simulink model "sampleModel84"  (Simulink 9.1)
settings: Solver=VariableStepAuto  StartTime=0.0  StopTime=10.0  RelTol=1e-3
undefined symbols (not defined in the file): DiscIntNeverNeededParam, Newton, Raphson
libraries: simulink x55
(part 2 of 2)

== system sampleModel84/cfblk150 ==
  cfblk1 : Inport
  cfblk8 : Inport  Port=2
  Action Port : ActionPort  ActionType=then
  cfblk3 : simulink/Continuous/PID Controller  Controller=PID  TimeDomain=Discrete-time  SampleTime=-1  IntegratorMethod=Forward Euler  FilterMethod=Forward Euler  Form=Parallel  UseFilter=on  ControllerParametersSource=internal  P=1  I=1  D=0  N=100  InitialConditionSource=internal  InitialConditionForIntegrator=0  InitialConditionForFilter=0  ExternalReset=none  LimitOutput=off  UpperSaturationLimit=inf  LowerSaturationLimit=-inf  LinearizeAsGain=off  AntiWindupMode=none  Kb=1  TrackingMode=off  Kt=1  PParamMin=[]  PParamMax=[]  IParamMin=[]  IParamMax=[]  DParamMin=[]  DParamMax=[]  NParamMin=[]  NParamMax=[]  KbParamMin=[]  KbParamMax=[]  KtParamMin=[]  KtParamMax=[]  POutMin=[]  POutMax=[]  IOutMin=[]  IOutMax=[]  DOutMin=[]  DOutMax=[]  NOutMin=[]  NOutMax=[]  KbOutMin=[]  KbOutMax=[]  KtOutMin=[]  KtOutMax=[]  IntegratorOutMin=[]  IntegratorOutMax=[]  FilterOutMin=[]  FilterOutMax=[]  SumOutMin=[]  SumOutMax=[]  SumI1OutMin=[]  SumI1OutMax=[]  SumI2OutMin=[]  SumI2OutMax=[]  SumI3OutMin=[]  SumI3OutMax=[]  SumDOutMin=[]  SumDOutMax=[]  SaturationOutMin=[]  SaturationOutMax=[]  IntegratorContinuousStateAttributes=''  IntegratorStateMustResolveToSignalObject=off  IntegratorRTWStateStorageClass=Auto  FilterContinuousStateAttributes=''  FilterStateMustResolveToSignalObject=off  FilterRTWStateStorageClass=Auto  DifferentiatorICPrevScaledInput=0  DifferentiatorOutMin=[]  DifferentiatorOutMax=[]  FilterDiffOutCoefMin=[]  FilterDiffOutCoefMax=[]  SumDenOutMin=[]  SumDenOutMax=[]  SumNumOutMin=[]  SumNumOutMax=[]  ReciprocalOutMin=[]  ReciprocalOutMax=[]  DivideOutMin=[]  DivideOutMax=[]  TunerSelectOption=Transfer Function Based (PID Tuner App)
  cfblk4 : Trigonometry
  cfblk5 : UnaryMinus
  cfblk6 : Sqrt  Operator=rSqrt  AlgorithmType=Newton-Raphson  SaturateOnIntegerOverflow=on
  cfblk7 : Subsystem
  cfblk2 : Outport
  cfblk9 : Outport  Port=2
  cfblk10 : Outport  Port=3
  wires:
  cfblk1/1 -> cfblk5/1
  cfblk4/1 -> cfblk3/1, cfblk9/1
  cfblk5/1 -> cfblk4/1
  cfblk8/1 -> cfblk2/1
  cfblk6/1 -> cfblk10/1
  cfblk7/1(cfblk2) -> cfblk6/1
  cfblk3/1 -> cfblk7/1(cfblk1)

== system sampleModel84/cfblk151 ==
  cfblk1 : Inport
  cfblk8 : Inport  Port=2
  cfblk9 : Inport  Port=3
  Action Port : ActionPort  ActionType=else
  cfblk10 : Delay
  cfblk3 : Delay  DelayLengthSource=Input port
      settings: InputPortMap=u0,p1
  cfblk4 : simulink/Discrete/Transfer Fcn Lead or Lag  PoleZ=0.95  ZeroZ=0.75  ICPrevOutput=0.0  ICPrevInput=0.0  DoSatur=off
      settings: SourceProductName=Simulink  SourceProductBaseCode=SL
  cfblk5 : DotProduct  InputSameDT=on  OutDataTypeStr=Inherit: Inherit via internal rule
  cfblk6 : Bias  Bias=[-271351723.485476]
  cfblk7 : Subsystem
  cfblk2 : Outport
  wires:
  cfblk9/1 -> cfblk4/1
  cfblk3/1 -> cfblk7/1(cfblk1)
  cfblk1/1 -> cfblk3/1
  cfblk6/1 -> cfblk2/1
  cfblk7/1(cfblk2) -> cfblk5/1
  cfblk8/1 -> cfblk5/2
  cfblk4/1 -> cfblk6/1
  cfblk5/1 -> cfblk10/1
  cfblk10/1 -> cfblk3/2

== system sampleModel84/cfblk98 ==
  cfblk1 : Inport
  cfblk2 : Outport
  wires:
  cfblk1/1 -> cfblk2/1

== system sampleModel84/cfblk99 ==
  cfblk1 : Inport
  cfblk2 : Outport
  wires:
  cfblk1/1 -> cfblk2/1

== system sampleModel84/cfblk134/cfblk11 ==
  cfblk1 : Inport
  cfblk2 : Outport
  wires:
  cfblk1/1 -> cfblk2/1

== system sampleModel84/cfblk134/cfblk12 ==
  cfblk1 : Inport
  cfblk2 : Outport
  wires:
  cfblk1/1 -> cfblk2/1

== system sampleModel84/cfblk134/cfblk13 ==
  cfblk1 : Inport
  cfblk2 : Outport
  wires:
  cfblk1/1 -> cfblk2/1

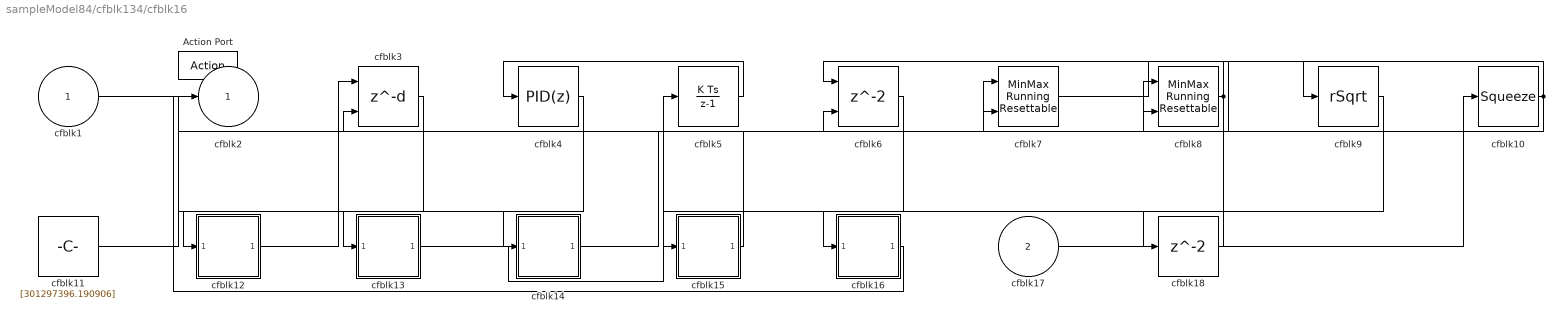
== system sampleModel84/cfblk134/cfblk16 ==
  cfblk1 : Inport
  cfblk17 : Inport  Port=2
  Action Port : ActionPort  ActionType=then
  cfblk10 : Squeeze
  cfblk11 : Constant  Value=[301297396.190906]  SampleTime=1
  cfblk12 : Subsystem
  cfblk13 : Subsystem
  cfblk14 : Subsystem
  cfblk15 : Subsystem
  cfblk16 : Subsystem
  cfblk18 : Delay
  cfblk3 : Delay  DelayLengthSource=Input port
      settings: InputPortMap=u0,p1
  cfblk4 : simulink/Continuous/PID Controller  Controller=PID  TimeDomain=Discrete-time  SampleTime=-1  IntegratorMethod=Forward Euler  FilterMethod=Forward Euler  Form=Parallel  UseFilter=on  ControllerParametersSource=internal  P=1  I=1  D=0  N=100  InitialConditionSource=internal  InitialConditionForIntegrator=0  InitialConditionForFilter=0  ExternalReset=none  LimitOutput=off  UpperSaturationLimit=inf  LowerSaturationLimit=-inf  LinearizeAsGain=off  AntiWindupMode=none  Kb=1  TrackingMode=off  Kt=1  PParamMin=[]  PParamMax=[]  IParamMin=[]  IParamMax=[]  DParamMin=[]  DParamMax=[]  NParamMin=[]  NParamMax=[]  KbParamMin=[]  KbParamMax=[]  KtParamMin=[]  KtParamMax=[]  POutMin=[]  POutMax=[]  IOutMin=[]  IOutMax=[]  DOutMin=[]  DOutMax=[]  NOutMin=[]  NOutMax=[]  KbOutMin=[]  KbOutMax=[]  KtOutMin=[]  KtOutMax=[]  IntegratorOutMin=[]  IntegratorOutMax=[]  FilterOutMin=[]  FilterOutMax=[]  SumOutMin=[]  SumOutMax=[]  SumI1OutMin=[]  SumI1OutMax=[]  SumI2OutMin=[]  SumI2OutMax=[]  SumI3OutMin=[]  SumI3OutMax=[]  SumDOutMin=[]  SumDOutMax=[]  SaturationOutMin=[]  SaturationOutMax=[]  IntegratorContinuousStateAttributes=''  IntegratorStateMustResolveToSignalObject=off  IntegratorRTWStateStorageClass=Auto  FilterContinuousStateAttributes=''  FilterStateMustResolveToSignalObject=off  FilterRTWStateStorageClass=Auto  DifferentiatorICPrevScaledInput=0  DifferentiatorOutMin=[]  DifferentiatorOutMax=[]  FilterDiffOutCoefMin=[]  FilterDiffOutCoefMax=[]  SumDenOutMin=[]  SumDenOutMax=[]  SumNumOutMin=[]  SumNumOutMax=[]  ReciprocalOutMin=[]  ReciprocalOutMax=[]  DivideOutMin=[]  DivideOutMax=[]  TunerSelectOption=Transfer Function Based (PID Tuner App)
  cfblk5 : DiscreteIntegrator  SampleTime=-1  ICPrevOutput=DiscIntNeverNeededParam  ICPrevScaledInput=DiscIntNeverNeededParam
  cfblk6 : Delay  ShowEnablePort=on
      settings: InputPortMap=u0,e6
  cfblk7 : simulink/Math Operations/MinMax Running Resettable  Function=min  vinit=0.0
  cfblk8 : simulink/Math Operations/MinMax Running Resettable  Function=min  vinit=0.0
  cfblk9 : Sqrt  Operator=rSqrt  AlgorithmType=Newton-Raphson  SaturateOnIntegerOverflow=on
  cfblk2 : Outport
  wires:
  cfblk4/1 -> cfblk12/1(cfblk1)
  cfblk13/1(cfblk2) -> cfblk5/1
  cfblk16/1(cfblk2) -> cfblk2/1
  cfblk9/1 -> cfblk15/1(cfblk1)
  cfblk8/1 -> cfblk6/1, cfblk18/1
  cfblk15/1(cfblk2) -> cfblk3/2
  cfblk1/1 -> cfblk14/1(cfblk1)
  cfblk10/1 -> cfblk7/1, cfblk6/2
  cfblk7/1 -> cfblk9/1
  cfblk3/1 -> cfblk13/1(cfblk1)
  cfblk17/1 -> cfblk10/1
  cfblk5/1 -> cfblk4/1
  cfblk14/1(cfblk2) -> cfblk7/2
  cfblk6/1 -> cfblk16/1(cfblk1)
  cfblk11/1 -> cfblk8/1
  cfblk12/1(cfblk2) -> cfblk8/2
  cfblk18/1 -> cfblk3/1

== system sampleModel84/cfblk134/cfblk17 ==
  cfblk1 : Inport
  cfblk8 : Inport  Port=2
  cfblk9 : Inport  Port=3
  Action Port : ActionPort  ActionType=else
  cfblk3 : simulink/Discrete/Transfer Fcn Real Zero  ZeroZ=0.75  ICPrevInput=0.0  DoSatur=off
      settings: SourceProductName=Simulink  SourceProductBaseCode=SL
  cfblk4 : Reshape
  cfblk5 : MinMax  Function=max  Inputs=3
  cfblk6 : Assignment  DiagnosticForDimensions=Warning  IndexOptions=Index vector (dialog)  Indices=1  OutputSizes=1
  cfblk7 : Polyval  Coefs=[ +2.081618890e-019, -1.441693666e-014, +4.719686976e-010, -8.536869453e-006, +1.621573104e-001, -8.087801117e+001 ]
  cfblk2 : Outport
  wires:
  cfblk1/1 -> cfblk3/1
  cfblk7/1 -> cfblk6/1
  cfblk8/1 -> cfblk4/1, cfblk5/3
  cfblk9/1 -> cfblk7/1
  cfblk3/1 -> cfblk6/2
  cfblk6/1 -> cfblk5/1
  cfblk4/1 -> cfblk2/1, cfblk5/2

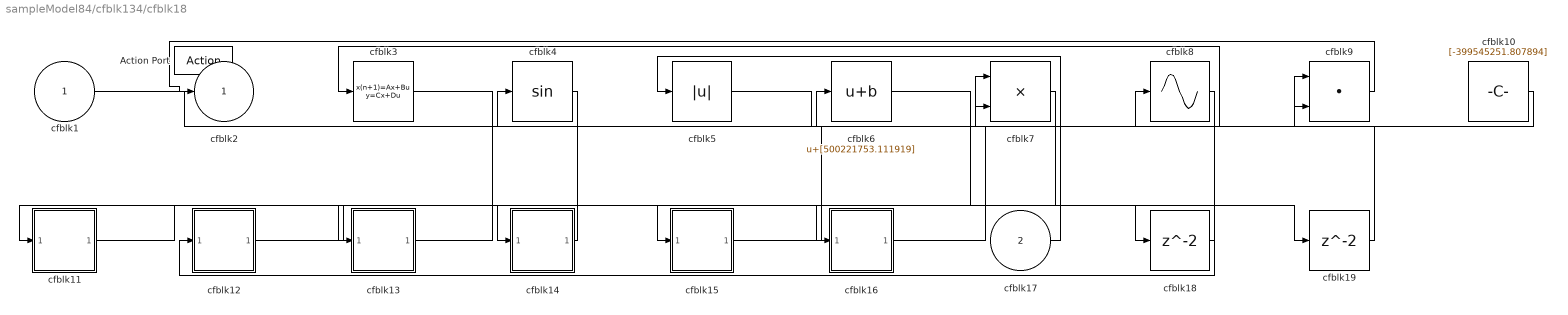
== system sampleModel84/cfblk134/cfblk18 ==
  cfblk1 : Inport
  cfblk17 : Inport  Port=2
  Action Port : ActionPort  ActionType=then
  cfblk10 : Constant  Value=[-399545251.807894]  SampleTime=1
  cfblk11 : Subsystem
  cfblk12 : Subsystem
  cfblk13 : Subsystem
  cfblk14 : Subsystem
  cfblk15 : Subsystem
  cfblk16 : Subsystem
  cfblk18 : Delay
  cfblk19 : Delay
  cfblk3 : DiscreteStateSpace  SampleTime=-1
  cfblk4 : Trigonometry
  cfblk5 : Abs
  cfblk6 : Bias  Bias=[500221753.111919]
  cfblk7 : Product  Inputs=**
  cfblk8 : Sin  TimeSource=Use external signal  SampleTime=0
  cfblk9 : DotProduct  InputSameDT=on  OutDataTypeStr=Inherit: Inherit via internal rule
  cfblk2 : Outport
  wires:
  cfblk1/1 -> cfblk7/1
  cfblk7/1 -> cfblk15/1(cfblk1)
  cfblk17/1 -> cfblk5/1
  cfblk8/1 -> cfblk12/1(cfblk1)
  cfblk12/1(cfblk2) -> cfblk14/1(cfblk1)
  cfblk9/1 -> cfblk2/1
  cfblk15/1(cfblk2) -> cfblk8/1
  cfblk10/1 -> cfblk3/1
  cfblk3/1 -> cfblk16/1(cfblk1)
  cfblk14/1(cfblk2) -> cfblk11/1(cfblk1)
  cfblk13/1(cfblk2) -> cfblk6/1
  cfblk4/1 -> cfblk13/1(cfblk1)
  cfblk16/1(cfblk2) -> cfblk9/1
  cfblk5/1 -> cfblk9/2
  cfblk11/1(cfblk2) -> cfblk18/1
  cfblk18/1 -> cfblk7/2
  cfblk6/1 -> cfblk19/1
  cfblk19/1 -> cfblk4/1

== system sampleModel84/cfblk134/cfblk19 ==
  cfblk1 : Inport
  Action Port : ActionPort  ActionType=else
  cfblk10 : Subsystem
  cfblk12 : Delay
  cfblk3 : simulink/Discrete/Difference  ICPrevInput=0.0  OutMin=[]  OutMax=[]  OutDataTypeStr=Inherit: Inherit via back propagation  OutDataType=fixdt(1, 16)  OutScaling=2^-10  DoSatur=off
  cfblk4 : simulink/Discrete/Transfer Fcn Real Zero  ZeroZ=0.75  ICPrevInput=0.0  DoSatur=off
      settings: SourceProductName=Simulink  SourceProductBaseCode=SL
  cfblk5 : Reshape
  cfblk6 : Polyval  Coefs=[ +2.081618890e-019, -1.441693666e-014, +4.719686976e-010, -8.536869453e-006, +1.621573104e-001, -8.087801117e+001 ]
  cfblk7 : Constant  Value=[-872675148.668030]  SampleTime=1
  cfblk8 : Subsystem
  cfblk9 : Subsystem
  cfblk2 : Outport
  cfblk11 : Outport  Port=2
  wires:
  cfblk5/1 -> cfblk8/1(cfblk1)
  cfblk6/1 -> cfblk9/1(cfblk1)
  cfblk1/1 -> cfblk3/1
  cfblk10/1(cfblk2) -> cfblk5/1
  cfblk8/1(cfblk2) -> cfblk11/1
  cfblk7/1 -> cfblk2/1
  cfblk4/1 -> cfblk10/1(cfblk1)
  cfblk3/1 -> cfblk4/1
  cfblk9/1(cfblk2) -> cfblk12/1
  cfblk12/1 -> cfblk6/1

== system sampleModel84/cfblk135/cfblk9 ==
  cfblk1 : Inport
  cfblk2 : Outport
  wires:
  cfblk1/1 -> cfblk2/1

== system sampleModel84/cfblk136/cfblk10 ==
  cfblk1 : Inport
  cfblk2 : Outport
  wires:
  cfblk1/1 -> cfblk2/1

== system sampleModel84/cfblk136/cfblk8 ==
  cfblk1 : Inport
  cfblk2 : Outport
  wires:
  cfblk1/1 -> cfblk2/1

== system sampleModel84/cfblk136/cfblk9 ==
  cfblk1 : Inport
  cfblk2 : Outport
  wires:
  cfblk1/1 -> cfblk2/1

== system sampleModel84/cfblk138/cfblk10 ==
  cfblk1 : Inport
  cfblk2 : Outport
  wires:
  cfblk1/1 -> cfblk2/1

== system sampleModel84/cfblk138/cfblk8 ==
  cfblk1 : Inport
  cfblk2 : Outport
  wires:
  cfblk1/1 -> cfblk2/1

== system sampleModel84/cfblk138/cfblk9 ==
  cfblk1 : Inport
  cfblk2 : Outport
  wires:
  cfblk1/1 -> cfblk2/1

== system sampleModel84/cfblk139/cfblk10 ==
  cfblk1 : Inport
  cfblk2 : Outport
  wires:
  cfblk1/1 -> cfblk2/1

== system sampleModel84/cfblk139/cfblk13 ==
  cfblk1 : Inport
  cfblk11 : Inport  Port=2
  cfblk12 : Inport  Port=3
  cfblk13 : Inport  Port=4
  cfblk14 : Inport  Port=5
  Action Port : ActionPort  ActionType=then
  cfblk10 : Subsystem
  cfblk3 : DiscreteTransferFcn
  cfblk4 : Squeeze
  cfblk5 : Sum  Inputs=+-
  cfblk6 : Sum  Inputs=+-
  cfblk7 : Sum  Inputs=|++
  cfblk8 : Product  Inputs=**
  cfblk9 : Constant  Value=[-663658281.904295]  SampleTime=1
  cfblk2 : Outport
  wires:
  cfblk1/1 -> cfblk2/1
  cfblk8/1 -> cfblk10/1(cfblk1)
  cfblk10/1(cfblk2) -> cfblk4/1
  cfblk3/1 -> cfblk7/1
  cfblk4/1 -> cfblk5/1
  cfblk11/1 -> cfblk6/1
  cfblk14/1 -> cfblk3/1
  cfblk6/1 -> cfblk7/2
  cfblk12/1 -> cfblk6/2
  cfblk7/1 -> cfblk8/1
  cfblk9/1 -> cfblk8/2
  cfblk13/1 -> cfblk5/2

== system sampleModel84/cfblk139/cfblk14 ==
  cfblk1 : Inport
  cfblk11 : Inport  Port=2
  cfblk12 : Inport  Port=3
  Action Port : ActionPort  ActionType=else
  cfblk10 : Subsystem
  cfblk3 : simulink/Discrete/Difference  ICPrevInput=0.0  OutMin=[]  OutMax=[]  OutDataTypeStr=Inherit: Inherit via back propagation  OutDataType=fixdt(1, 16)  OutScaling=2^-10  DoSatur=off
  cfblk4 : DiscreteStateSpace  SampleTime=-1
  cfblk5 : simulink/Discrete/Difference  ICPrevInput=0.0  OutMin=[]  OutMax=[]  OutDataTypeStr=Inherit: Inherit via back propagation  OutDataType=fixdt(1, 16)  OutScaling=2^-10  DoSatur=off
  cfblk6 : Math  Operator=conj  SaturateOnIntegerOverflow=on
  cfblk7 : Sum  Inputs=+
  cfblk8 : Constant  Value=[-583417160.658868]  SampleTime=1
  cfblk9 : Subsystem
  cfblk2 : Outport
  wires:
  cfblk1/1 -> cfblk9/1(cfblk1)
  cfblk10/1(cfblk2) -> cfblk5/1
  cfblk9/1(cfblk2) -> cfblk10/1(cfblk1)
  cfblk12/1 -> cfblk2/1
  cfblk8/1 -> cfblk6/1
  cfblk6/1 -> cfblk3/1
  cfblk3/1 -> cfblk7/1
  cfblk11/1 -> cfblk4/1

== system sampleModel84/cfblk139/cfblk8 ==
  cfblk1 : Inport
  cfblk2 : Outport
  wires:
  cfblk1/1 -> cfblk2/1

== system sampleModel84/cfblk139/cfblk9 ==
  cfblk1 : Inport
  cfblk2 : Outport
  wires:
  cfblk1/1 -> cfblk2/1

== system sampleModel84/cfblk140/cfblk11 ==
  cfblk1 : Inport
  cfblk2 : Outport
  wires:
  cfblk1/1 -> cfblk2/1

== system sampleModel84/cfblk140/cfblk12 ==
  cfblk1 : Inport
  cfblk2 : Outport
  wires:
  cfblk1/1 -> cfblk2/1

== system sampleModel84/cfblk140/cfblk13 ==
  cfblk1 : Inport
  cfblk2 : Outport
  wires:
  cfblk1/1 -> cfblk2/1

== system sampleModel84/cfblk140/cfblk14 ==
  cfblk1 : Inport
  cfblk2 : Outport
  wires:
  cfblk1/1 -> cfblk2/1

== system sampleModel84/cfblk141/cfblk11 ==
  cfblk1 : Inport
  cfblk2 : Outport
  wires:
  cfblk1/1 -> cfblk2/1

== system sampleModel84/cfblk141/cfblk12 ==
  cfblk1 : Inport
  cfblk2 : Outport
  wires:
  cfblk1/1 -> cfblk2/1

== system sampleModel84/cfblk141/cfblk13 ==
  cfblk1 : Inport
  cfblk2 : Outport
  wires:
  cfblk1/1 -> cfblk2/1

== system sampleModel84/cfblk141/cfblk14 ==
  cfblk1 : Inport
  cfblk2 : Outport
  wires:
  cfblk1/1 -> cfblk2/1

== system sampleModel84/cfblk142/cfblk5 ==
  cfblk1 : Inport
  cfblk2 : Outport
  wires:
  cfblk1/1 -> cfblk2/1

== system sampleModel84/cfblk142/cfblk6 ==
  cfblk1 : Inport
  cfblk2 : Outport
  wires:
  cfblk1/1 -> cfblk2/1

== system sampleModel84/cfblk142/cfblk7 ==
  cfblk1 : Inport
  cfblk2 : Outport
  wires:
  cfblk1/1 -> cfblk2/1

== system sampleModel84/cfblk143/cfblk11 ==
  cfblk1 : Inport
  cfblk2 : Outport
  wires:
  cfblk1/1 -> cfblk2/1

== system sampleModel84/cfblk143/cfblk12 ==
  cfblk1 : Inport
  cfblk2 : Outport
  wires:
  cfblk1/1 -> cfblk2/1

== system sampleModel84/cfblk143/cfblk13 ==
  cfblk1 : Inport
  cfblk2 : Outport
  wires:
  cfblk1/1 -> cfblk2/1

== system sampleModel84/cfblk143/cfblk14 ==
  cfblk1 : Inport
  cfblk2 : Outport
  wires:
  cfblk1/1 -> cfblk2/1

== system sampleModel84/cfblk144/cfblk12 ==
  cfblk1 : Inport
  cfblk2 : Outport
  wires:
  cfblk1/1 -> cfblk2/1

== system sampleModel84/cfblk144/cfblk13 ==
  cfblk1 : Inport
  cfblk2 : Outport
  wires:
  cfblk1/1 -> cfblk2/1

== system sampleModel84/cfblk144/cfblk14 ==
  cfblk1 : Inport
  cfblk2 : Outport
  wires:
  cfblk1/1 -> cfblk2/1

== system sampleModel84/cfblk144/cfblk15 ==
  cfblk1 : Inport
  cfblk2 : Outport
  wires:
  cfblk1/1 -> cfblk2/1

== system sampleModel84/cfblk144/cfblk16 ==
  cfblk1 : Inport
  cfblk2 : Outport
  wires:
  cfblk1/1 -> cfblk2/1

== system sampleModel84/cfblk145/cfblk6 ==
  cfblk1 : Inport
  cfblk2 : Outport
  wires:
  cfblk1/1 -> cfblk2/1

== system sampleModel84/cfblk145/cfblk7 ==
  cfblk1 : Inport
  cfblk2 : Outport
  wires:
  cfblk1/1 -> cfblk2/1

== system sampleModel84/cfblk145/cfblk8 ==
  cfblk1 : Inport
  cfblk2 : Outport
  wires:
  cfblk1/1 -> cfblk2/1

== system sampleModel84/cfblk145/cfblk9 ==
  cfblk1 : Inport
  cfblk2 : Outport
  wires:
  cfblk1/1 -> cfblk2/1

== system sampleModel84/cfblk146/cfblk11 ==
  cfblk1 : Inport
  cfblk2 : Outport
  wires:
  cfblk1/1 -> cfblk2/1

== system sampleModel84/cfblk146/cfblk12 ==
  cfblk1 : Inport
  cfblk2 : Outport
  wires:
  cfblk1/1 -> cfblk2/1

== system sampleModel84/cfblk146/cfblk13 ==
  cfblk1 : Inport
  cfblk2 : Outport
  wires:
  cfblk1/1 -> cfblk2/1

== system sampleModel84/cfblk146/cfblk14 ==
  cfblk1 : Inport
  cfblk2 : Outport
  wires:
  cfblk1/1 -> cfblk2/1

== system sampleModel84/cfblk146/cfblk15 ==
  cfblk1 : Inport
  cfblk2 : Outport
  wires:
  cfblk1/1 -> cfblk2/1

== system sampleModel84/cfblk147/cfblk5 ==
  cfblk1 : Inport
  cfblk2 : Outport
  wires:
  cfblk1/1 -> cfblk2/1

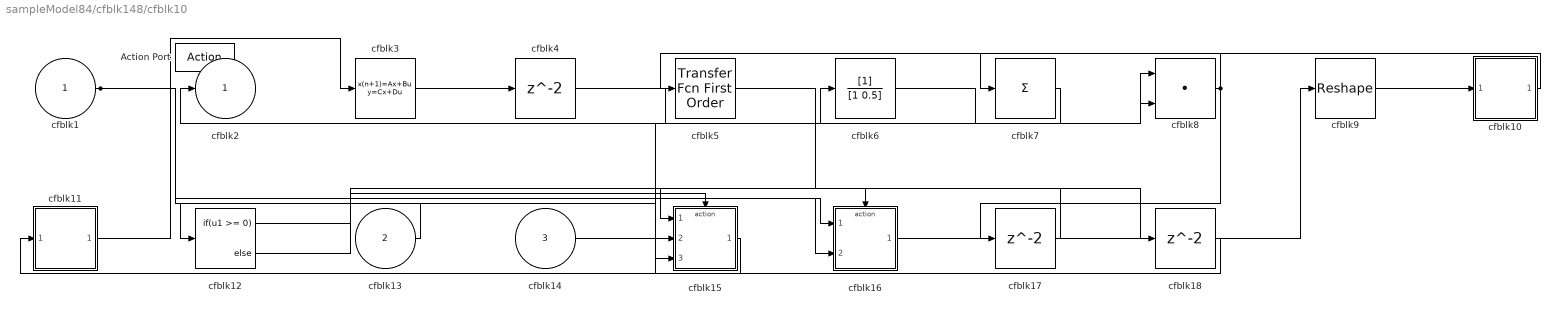
== system sampleModel84/cfblk148/cfblk10 ==
  cfblk1 : Inport
  cfblk13 : Inport  Port=2
  cfblk14 : Inport  Port=3
  Action Port : ActionPort  ActionType=then
  cfblk10 : Subsystem
  cfblk11 : Subsystem
  cfblk12 : If  IfExpression=u1 >= 0  SampleTime=1
  cfblk15 : Subsystem  TreatAsAtomicUnit=on
  cfblk16 : Subsystem  TreatAsAtomicUnit=on
  cfblk17 : Delay
  cfblk18 : Delay
  cfblk3 : DiscreteStateSpace  SampleTime=-1
  cfblk4 : Delay
  cfblk5 : simulink/Discrete/Transfer Fcn First Order  PoleZ=0.95  ICPrevOutput=0.0  DoSatur=off
      settings: SourceProductName=Simulink
  cfblk6 : DiscreteFilter
  cfblk7 : Sum  Inputs=+
  cfblk8 : DotProduct  InputSameDT=on  OutDataTypeStr=Inherit: Inherit via internal rule
  cfblk9 : Reshape
  cfblk2 : Outport
  wires:
  cfblk10/1(cfblk2) -> cfblk7/1
  cfblk8/1 -> cfblk5/1, cfblk17/1
  cfblk4/1 -> cfblk8/1
  cfblk13/1 -> cfblk12/1
  cfblk7/1 -> cfblk2/1
  cfblk3/1 -> cfblk4/1
  cfblk15/1(cfblk2) -> cfblk11/1(cfblk1)
  cfblk9/1 -> cfblk10/1(cfblk1)
  cfblk16/1(cfblk2) -> cfblk9/1
  cfblk11/1(cfblk2) -> cfblk3/1
  cfblk14/1 -> cfblk6/1
  cfblk6/1 -> cfblk8/2
  cfblk1/1 -> cfblk16/1(cfblk1), cfblk15/3(cfblk15), cfblk16/2(cfblk11)
  cfblk12/1 -> cfblk15/Action
  cfblk12/2 -> cfblk16/Action
  cfblk17/1 -> cfblk15/1(cfblk1)
  cfblk5/1 -> cfblk18/1
  cfblk18/1 -> cfblk15/2(cfblk14)

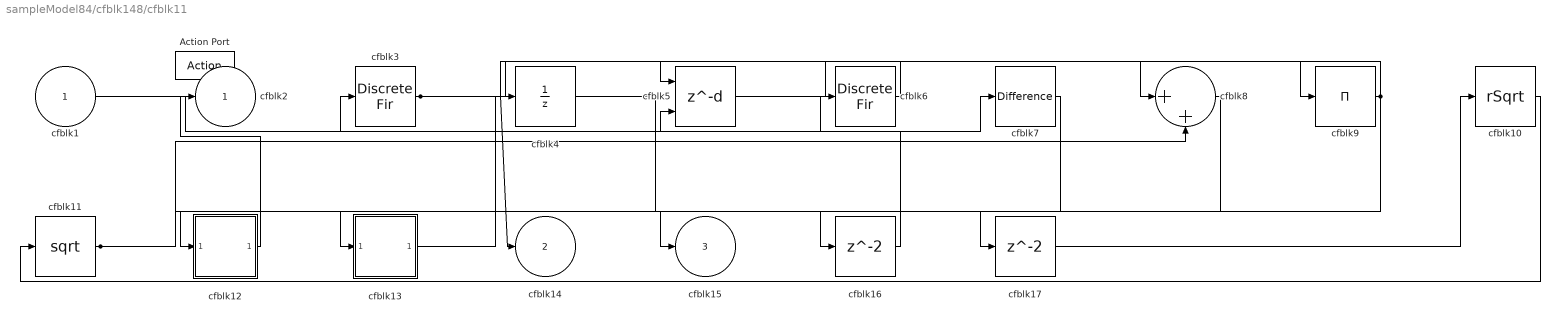
== system sampleModel84/cfblk148/cfblk11 ==
  cfblk1 : Inport
  Action Port : ActionPort  ActionType=else
  cfblk10 : Sqrt  Operator=rSqrt  AlgorithmType=Newton-Raphson  SaturateOnIntegerOverflow=on
  cfblk11 : Sqrt  SaturateOnIntegerOverflow=on
  cfblk12 : Subsystem
  cfblk13 : Subsystem
  cfblk16 : Delay
  cfblk17 : Delay
  cfblk3 : DiscreteFir
  cfblk4 : UnitDelay  SampleTime=-1
  cfblk5 : Delay  DelayLengthSource=Input port
      settings: InputPortMap=u0,p1
  cfblk6 : DiscreteFir
  cfblk7 : simulink/Discrete/Difference  ICPrevInput=0.0  OutMin=[]  OutMax=[]  OutDataTypeStr=Inherit: Inherit via back propagation  OutDataType=fixdt(1, 16)  OutScaling=2^-10  DoSatur=off
  cfblk8 : Sum  Inputs=|++
  cfblk9 : Product  Inputs=*
  cfblk2 : Outport
  cfblk14 : Outport  Port=2
  cfblk15 : Outport  Port=3
  wires:
  cfblk5/1 -> cfblk8/1
  cfblk1/1 -> cfblk7/1
  cfblk12/1(cfblk2) -> cfblk2/1
  cfblk10/1 -> cfblk11/1
  cfblk11/1 -> cfblk8/2, cfblk17/1
  cfblk3/1 -> cfblk14/1, cfblk9/1, cfblk5/2
  cfblk6/1 -> cfblk5/1
  cfblk9/1 -> cfblk12/1(cfblk1), cfblk4/1
  cfblk7/1 -> cfblk13/1(cfblk1)
  cfblk13/1(cfblk2) -> cfblk6/1
  cfblk8/1 -> cfblk15/1
  cfblk4/1 -> cfblk16/1
  cfblk16/1 -> cfblk3/1
  cfblk17/1 -> cfblk10/1

== system sampleModel84/cfblk148/cfblk5 ==
  cfblk1 : Inport
  cfblk2 : Outport
  wires:
  cfblk1/1 -> cfblk2/1

== system sampleModel84/cfblk148/cfblk6 ==
  cfblk1 : Inport
  cfblk2 : Outport
  wires:
  cfblk1/1 -> cfblk2/1

== system sampleModel84/cfblk148/cfblk7 ==
  cfblk1 : Inport
  cfblk2 : Outport
  wires:
  cfblk1/1 -> cfblk2/1

== system sampleModel84/cfblk148/cfblk8 ==
  cfblk1 : Inport
  cfblk2 : Outport
  wires:
  cfblk1/1 -> cfblk2/1

== system sampleModel84/cfblk149/cfblk10 ==
  cfblk1 : Inport
  cfblk2 : Outport
  wires:
  cfblk1/1 -> cfblk2/1

== system sampleModel84/cfblk149/cfblk11 ==
  cfblk1 : Inport
  cfblk2 : Outport
  wires:
  cfblk1/1 -> cfblk2/1

== system sampleModel84/cfblk149/cfblk12 ==
  cfblk1 : Inport
  cfblk2 : Outport
  wires:
  cfblk1/1 -> cfblk2/1

== system sampleModel84/cfblk149/cfblk8 ==
  cfblk1 : Inport
  cfblk2 : Outport
  wires:
  cfblk1/1 -> cfblk2/1

== system sampleModel84/cfblk149/cfblk9 ==
  cfblk1 : Inport
  cfblk2 : Outport
  wires:
  cfblk1/1 -> cfblk2/1

== system sampleModel84/cfblk150/cfblk7 ==
  cfblk1 : Inport
  cfblk2 : Outport
  wires:
  cfblk1/1 -> cfblk2/1

== system sampleModel84/cfblk151/cfblk7 ==
  cfblk1 : Inport
  cfblk2 : Outport
  wires:
  cfblk1/1 -> cfblk2/1

== system sampleModel84/cfblk134/cfblk16/cfblk12 ==
  cfblk1 : Inport
  cfblk2 : Outport
  wires:
  cfblk1/1 -> cfblk2/1

== system sampleModel84/cfblk134/cfblk16/cfblk13 ==
  cfblk1 : Inport
  cfblk2 : Outport
  wires:
  cfblk1/1 -> cfblk2/1

== system sampleModel84/cfblk134/cfblk16/cfblk14 ==
  cfblk1 : Inport
  cfblk2 : Outport
  wires:
  cfblk1/1 -> cfblk2/1

== system sampleModel84/cfblk134/cfblk16/cfblk15 ==
  cfblk1 : Inport
  cfblk2 : Outport
  wires:
  cfblk1/1 -> cfblk2/1

== system sampleModel84/cfblk134/cfblk16/cfblk16 ==
  cfblk1 : Inport
  cfblk2 : Outport
  wires:
  cfblk1/1 -> cfblk2/1

== system sampleModel84/cfblk134/cfblk18/cfblk11 ==
  cfblk1 : Inport
  cfblk2 : Outport
  wires:
  cfblk1/1 -> cfblk2/1

== system sampleModel84/cfblk134/cfblk18/cfblk12 ==
  cfblk1 : Inport
  cfblk2 : Outport
  wires:
  cfblk1/1 -> cfblk2/1

== system sampleModel84/cfblk134/cfblk18/cfblk13 ==
  cfblk1 : Inport
  cfblk2 : Outport
  wires:
  cfblk1/1 -> cfblk2/1

== system sampleModel84/cfblk134/cfblk18/cfblk14 ==
  cfblk1 : Inport
  cfblk2 : Outport
  wires:
  cfblk1/1 -> cfblk2/1

== system sampleModel84/cfblk134/cfblk18/cfblk15 ==
  cfblk1 : Inport
  cfblk2 : Outport
  wires:
  cfblk1/1 -> cfblk2/1

== system sampleModel84/cfblk134/cfblk18/cfblk16 ==
  cfblk1 : Inport
  cfblk2 : Outport
  wires:
  cfblk1/1 -> cfblk2/1

== system sampleModel84/cfblk134/cfblk19/cfblk10 ==
  cfblk1 : Inport
  cfblk2 : Outport
  wires:
  cfblk1/1 -> cfblk2/1

== system sampleModel84/cfblk134/cfblk19/cfblk8 ==
  cfblk1 : Inport
  cfblk2 : Outport
  wires:
  cfblk1/1 -> cfblk2/1

== system sampleModel84/cfblk134/cfblk19/cfblk9 ==
  cfblk1 : Inport
  cfblk2 : Outport
  wires:
  cfblk1/1 -> cfblk2/1

== system sampleModel84/cfblk139/cfblk13/cfblk10 ==
  cfblk1 : Inport
  cfblk2 : Outport
  wires:
  cfblk1/1 -> cfblk2/1

== system sampleModel84/cfblk139/cfblk14/cfblk10 ==
  cfblk1 : Inport
  cfblk2 : Outport
  wires:
  cfblk1/1 -> cfblk2/1

== system sampleModel84/cfblk139/cfblk14/cfblk9 ==
  cfblk1 : Inport
  cfblk2 : Outport
  wires:
  cfblk1/1 -> cfblk2/1

== system sampleModel84/cfblk148/cfblk10/cfblk10 ==
  cfblk1 : Inport
  cfblk2 : Outport
  wires:
  cfblk1/1 -> cfblk2/1

== system sampleModel84/cfblk148/cfblk10/cfblk11 ==
  cfblk1 : Inport
  cfblk2 : Outport
  wires:
  cfblk1/1 -> cfblk2/1

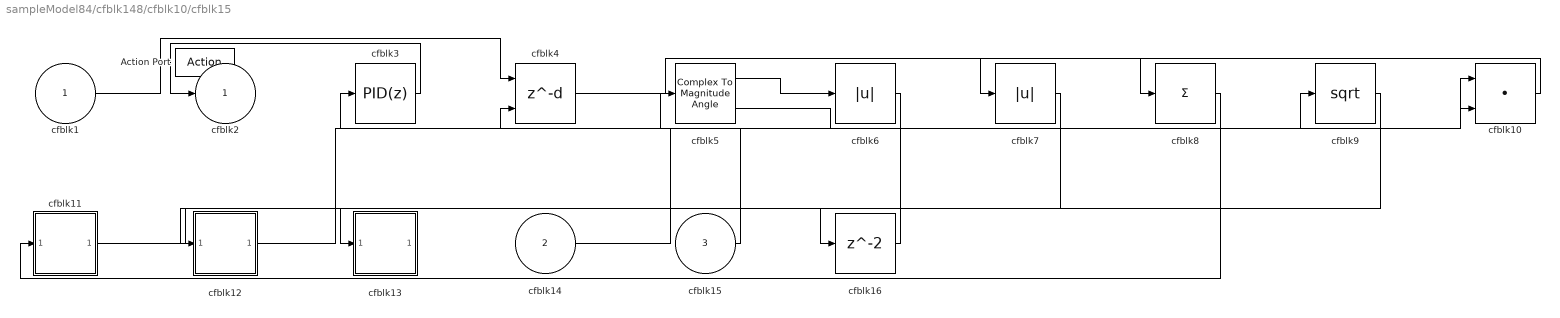
== system sampleModel84/cfblk148/cfblk10/cfblk15 ==
  cfblk1 : Inport
  cfblk14 : Inport  Port=2
  cfblk15 : Inport  Port=3
  Action Port : ActionPort  ActionType=then
  cfblk10 : DotProduct  InputSameDT=on  OutDataTypeStr=Inherit: Inherit via internal rule
  cfblk11 : Subsystem
  cfblk12 : Subsystem
  cfblk13 : Subsystem
  cfblk16 : Delay
  cfblk3 : simulink/Continuous/PID Controller  Controller=PID  TimeDomain=Discrete-time  SampleTime=-1  IntegratorMethod=Forward Euler  FilterMethod=Forward Euler  Form=Parallel  UseFilter=on  ControllerParametersSource=internal  P=1  I=1  D=0  N=100  InitialConditionSource=internal  InitialConditionForIntegrator=0  InitialConditionForFilter=0  ExternalReset=none  LimitOutput=off  UpperSaturationLimit=inf  LowerSaturationLimit=-inf  LinearizeAsGain=off  AntiWindupMode=none  Kb=1  TrackingMode=off  Kt=1  PParamMin=[]  PParamMax=[]  IParamMin=[]  IParamMax=[]  DParamMin=[]  DParamMax=[]  NParamMin=[]  NParamMax=[]  KbParamMin=[]  KbParamMax=[]  KtParamMin=[]  KtParamMax=[]  POutMin=[]  POutMax=[]  IOutMin=[]  IOutMax=[]  DOutMin=[]  DOutMax=[]  NOutMin=[]  NOutMax=[]  KbOutMin=[]  KbOutMax=[]  KtOutMin=[]  KtOutMax=[]  IntegratorOutMin=[]  IntegratorOutMax=[]  FilterOutMin=[]  FilterOutMax=[]  SumOutMin=[]  SumOutMax=[]  SumI1OutMin=[]  SumI1OutMax=[]  SumI2OutMin=[]  SumI2OutMax=[]  SumI3OutMin=[]  SumI3OutMax=[]  SumDOutMin=[]  SumDOutMax=[]  SaturationOutMin=[]  SaturationOutMax=[]  IntegratorContinuousStateAttributes=''  IntegratorStateMustResolveToSignalObject=off  IntegratorRTWStateStorageClass=Auto  FilterContinuousStateAttributes=''  FilterStateMustResolveToSignalObject=off  FilterRTWStateStorageClass=Auto  DifferentiatorICPrevScaledInput=0  DifferentiatorOutMin=[]  DifferentiatorOutMax=[]  FilterDiffOutCoefMin=[]  FilterDiffOutCoefMax=[]  SumDenOutMin=[]  SumDenOutMax=[]  SumNumOutMin=[]  SumNumOutMax=[]  ReciprocalOutMin=[]  ReciprocalOutMax=[]  DivideOutMin=[]  DivideOutMax=[]  TunerSelectOption=Transfer Function Based (PID Tuner App)
  cfblk4 : Delay  DelayLengthSource=Input port
      settings: InputPortMap=u0,p1
  cfblk5 : ComplexToMagnitudeAngle
  cfblk6 : Abs
  cfblk7 : Abs
  cfblk8 : Sum  Inputs=+
  cfblk9 : Sqrt  SaturateOnIntegerOverflow=on
  cfblk2 : Outport
  wires:
  cfblk15/1 -> cfblk3/1
  cfblk3/1 -> cfblk2/1
  cfblk8/1 -> cfblk11/1(cfblk1)
  cfblk11/1(cfblk2) -> cfblk13/1(cfblk1)
  cfblk10/1 -> cfblk7/1
  cfblk9/1 -> cfblk12/1(cfblk1)
  cfblk1/1 -> cfblk4/1
  cfblk5/1 -> cfblk6/1
  cfblk6/1 -> cfblk4/2
  cfblk14/1 -> cfblk10/1
  cfblk5/2 -> cfblk9/1
  cfblk4/1 -> cfblk8/1
  cfblk12/1(cfblk2) -> cfblk10/2
  cfblk7/1 -> cfblk16/1
  cfblk16/1 -> cfblk5/1

== system sampleModel84/cfblk148/cfblk10/cfblk16 ==
  cfblk1 : Inport
  cfblk11 : Inport  Port=2
  Action Port : ActionPort  ActionType=else
  cfblk10 : Subsystem
  cfblk12 : Delay
  cfblk3 : PermuteDimensions
  cfblk4 : simulink/Math Operations/MinMax Running Resettable  Function=min  vinit=0.0
  cfblk5 : Squeeze
  cfblk6 : Sum  Inputs=+
  cfblk7 : Constant  Value=[515722685.373145]  SampleTime=1
  cfblk8 : Subsystem
  cfblk9 : Subsystem
  cfblk2 : Outport
  wires:
  cfblk10/1(cfblk2) -> cfblk6/1
  cfblk11/1 -> cfblk3/1
  cfblk8/1(cfblk2) -> cfblk2/1
  cfblk4/1 -> cfblk9/1(cfblk1)
  cfblk3/1 -> cfblk10/1(cfblk1)
  cfblk6/1 -> cfblk5/1
  cfblk1/1 -> cfblk8/1(cfblk1)
  cfblk7/1 -> cfblk4/1
  cfblk9/1(cfblk2) -> cfblk12/1
  cfblk12/1 -> cfblk4/2

== system sampleModel84/cfblk148/cfblk11/cfblk12 ==
  cfblk1 : Inport
  cfblk2 : Outport
  wires:
  cfblk1/1 -> cfblk2/1

== system sampleModel84/cfblk148/cfblk11/cfblk13 ==
  cfblk1 : Inport
  cfblk2 : Outport
  wires:
  cfblk1/1 -> cfblk2/1

== system sampleModel84/cfblk148/cfblk10/cfblk15/cfblk11 ==
  cfblk1 : Inport
  cfblk2 : Outport
  wires:
  cfblk1/1 -> cfblk2/1

== system sampleModel84/cfblk148/cfblk10/cfblk15/cfblk12 ==
  cfblk1 : Inport
  cfblk2 : Outport
  wires:
  cfblk1/1 -> cfblk2/1

== system sampleModel84/cfblk148/cfblk10/cfblk15/cfblk13 ==
  cfblk1 : Inport
  cfblk2 : Outport
  wires:
  cfblk1/1 -> cfblk2/1

== system sampleModel84/cfblk148/cfblk10/cfblk16/cfblk10 ==
  cfblk1 : Inport
  cfblk2 : Outport
  wires:
  cfblk1/1 -> cfblk2/1

== system sampleModel84/cfblk148/cfblk10/cfblk16/cfblk8 ==
  cfblk1 : Inport
  cfblk2 : Outport
  wires:
  cfblk1/1 -> cfblk2/1

== system sampleModel84/cfblk148/cfblk10/cfblk16/cfblk9 ==
  cfblk1 : Inport
  cfblk2 : Outport
  wires:
  cfblk1/1 -> cfblk2/1
